simulink model "m_deadlogic01"  (Simulink 7.8)
settings: Solver=FixedStepDiscrete  StartTime=0.0  StopTime=10.0  FixedStep=Auto  RelTol=1e-3
libraries: simulink x2
settings Model: Creator=itoy  LastModifiedBy=itoy
settings DataIOCC: LimitDataPoints=off  SaveFormat=StructureWithTime  SaveOutput=off  SaveTime=off
settings OptimizationCC: OptimizeModelRefInitCode=on  LifeSpan=1
settings DebuggingCC: StrictBusMsg=Warning
settings RTWCC: SystemTargetFile=ert.tlc  GenCodeOnly=on  TemplateMakefile=ert_default_tmf  Description=Real-Time Workshop Embedded Coder  GenerateReport=on  ProcessScript=ert_make_rtw_hook  IncludeHyperlinkInReport=on  LaunchReport=on  GenerateTraceInfo=on  GenerateTraceReport=on  GenerateTraceReportSl=on  GenerateTraceReportSf=on  GenerateTraceReportEml=on
settings CodeAppCC: IgnoreCustomStorageClasses=off
settings ERTTargetCC: MultiwordLength=2048  GenerateSampleERTMain=on  ERTCustomFileTemplate=example_file_process.tlc  ConvertIfToSwitch=off  SuppressUnreachableDefaultCases=off

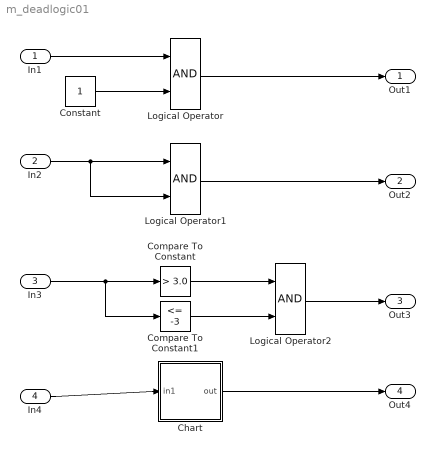
== system m_deadlogic01 ==
  In1 : Inport
  In2 : Inport  Port=2
  In3 : Inport  Port=3
  In4 : Inport  Port=4
  Chart : Stateflow chart  TreatAsAtomicUnit=on
  Compare To Constant : simulink/Logic and Bit Operations/Compare To Constant  relop=>  const=3.0  OutDataTypeStr=uint8
  Compare To Constant1 : simulink/Logic and Bit Operations/Compare To Constant  relop=<=  const=-3  OutDataTypeStr=uint8
  Constant : Constant
  Logical Operator : Logic  AllPortsSameDT=off  OutDataTypeStr=boolean
  Logical Operator1 : Logic  AllPortsSameDT=off  OutDataTypeStr=boolean
  Logical Operator2 : Logic  AllPortsSameDT=off  OutDataTypeStr=boolean
  Out1 : Outport
  Out2 : Outport  Port=2
  Out3 : Outport  Port=3
  Out4 : Outport  Port=4
  wires:
  In1/1 -> Logical Operator/1
  Constant/1 -> Logical Operator/2
  Logical Operator/1 -> Out1/1
  In2/1 -> Logical Operator1/1, Logical Operator1/2
  Logical Operator1/1 -> Out2/1
  In3/1 -> Compare To Constant/1, Compare To Constant1/1
  Compare To Constant/1 -> Logical Operator2/1
  Compare To Constant1/1 -> Logical Operator2/2
  Logical Operator2/1 -> Out3/1
  In4/1 -> Chart/1(in1)
  Chart/1(out) -> Out4/1

== stateflow chart Chart ==
  (default) -> (junction 3)
  (junction 3) -> (junction 4) [order 2]
  (junction 3) -> (junction 5) [order 1] : [in1 > 0 ]
  (junction 5) -> (junction 6) : {
      | out++;
      | }
  (junction 6) -> (junction 7) : [ in1 < -1]
  (junction 7) -> (junction 8) : {
      | out--;
      | }
  (junction 4) -> (junction 9) [order 1] : [ in1 < -1]
  (junction 9) -> (junction 10) : {
      | out--;
      | }
  (junction 4) -> (junction 11) [order 2]
  (junction 10) -> (junction 11)
  (junction 8) -> (junction 10)
  data: in1 input double; out output double
